simulink model "motor"  (Simulink 8.6)
settings: Solver=FixedStepDiscrete  StartTime=0.0  StopTime=inf  FixedStep=0.002  RelTol=1e-3
PostLoadFcn:
  | ,try, rti_mdl_postloadfcn(bdroot, 'UpdateModel', 160, 'rti1104'); catch, disp(lasterr); end,
undefined symbols (not defined in the file): DiscIntNeverNeededParam
(part 2 of 3)

== system motor/Chart/Open_Motor/sudu_PI ==
  In_ZV : Inport
  Discrete-Time Integrator : DiscreteIntegrator  ExternalReset=either  SampleTime=-1  SaturateOnIntegerOverflow=on  LimitOutput=on  UpperSaturationLimit=1000  LowerSaturationLimit=-1000  ICPrevOutput=DiscIntNeverNeededParam  ICPrevScaledInput=DiscIntNeverNeededParam
  Discrete-Time Integrator1 : DiscreteIntegrator  InitialConditionSetting=State (most efficient)  SampleTime=-1  ICPrevOutput=DiscIntNeverNeededParam  ICPrevScaledInput=DiscIntNeverNeededParam
  KD_KG : Gain  Gain=0
  KG_clc : DataStoreRead  DataStoreName=KG_clc
  Saturation : Saturate  UpperLimit=300  LowerLimit=-300
  Sum : Sum  Inputs=|+-
  Sum2 : Sum  Inputs=|+++
  ZV_KD : Gain  Gain=0.095
  ZV_KN : Gain  Gain=100
  ZV_Ki : Gain  Gain=0
  ZV_Kp : Gain  Gain=0.7
  ZV_Kp1 : Gain  Gain=0.001
  ZV_Kpt : Gain
  Out_ZV : Outport
  wires:
  ZV_Kpt/1 -> Sum2/2
  Discrete-Time Integrator/1 -> Sum2/1
  In_ZV/1 -> ZV_Kp/1
  ZV_Kp/1 -> ZV_Ki/1, ZV_Kp1/1, ZV_Kpt/1
  Sum2/1 -> Out_ZV/1
  ZV_Kp1/1 -> ZV_KD/1
  ZV_KD/1 -> Sum/1
  Sum/1 -> ZV_KN/1
  Discrete-Time Integrator1/1 -> Sum/2
  ZV_KN/1 -> Saturation/1, Discrete-Time Integrator1/1
  Saturation/1 -> KD_KG/1
  KD_KG/1 -> Sum2/3
  KG_clc/1 -> Discrete-Time Integrator/2
  ZV_Ki/1 -> Discrete-Time Integrator/1

== system motor/Chart/Showing/If Action Subsystem1 ==
  Action Port : ActionPort  ActionType=then
  Data Store Write : DataStoreWrite  DataStoreName=Angle_S
  Sine Wave : Sin  Frequency=pi/3
  wires:
  Sine Wave/1 -> Data Store Write/1

== system motor/Chart/Showing/If Action Subsystem2 ==
  Action Port : ActionPort  ActionType=elseif
  Data Store Write : DataStoreWrite  DataStoreName=Angle_S
  Sine Wave : Sin  Frequency=pi/4
  wires:
  Sine Wave/1 -> Data Store Write/1

== system motor/Chart/Showing/If Action Subsystem3 ==
  Action Port : ActionPort  ActionType=then
  Data Store Write : DataStoreWrite  DataStoreName=Angle_S
  Sine Wave : Sin  Frequency=pi/5
  wires:
  Sine Wave/1 -> Data Store Write/1

== system motor/Chart/Showing/If Action Subsystem4 ==
  Action Port : ActionPort  ActionType=elseif
  Data Store Write : DataStoreWrite  DataStoreName=Angle_S
  Sine Wave : Sin  Frequency=pi/6
  wires:
  Sine Wave/1 -> Data Store Write/1

== system motor/Chart/Showing/If Action Subsystem5 ==
  Action Port : ActionPort  ActionType=then
  Data Store Write : DataStoreWrite  DataStoreName=Angle_S
  Sine Wave : Sin  Frequency=pi/8
  wires:
  Sine Wave/1 -> Data Store Write/1

== system motor/Chart/Showing/If Action Subsystem6 ==
  Action Port : ActionPort  ActionType=elseif
  Data Store Write : DataStoreWrite  DataStoreName=Angle_S
  Sine Wave : Sin  Frequency=pi/10
  wires:
  Sine Wave/1 -> Data Store Write/1

== system motor/Chart/Showing/If Action Subsystem7 ==
  Action Port : ActionPort  ActionType=then
  Data Store Write : DataStoreWrite  DataStoreName=Angle_S
  Sine Wave : Sin  Frequency=pi/13
  wires:
  Sine Wave/1 -> Data Store Write/1

== system motor/Chart/Showing/If Action Subsystem8 ==
  Action Port : ActionPort  ActionType=elseif
  Data Store Write : DataStoreWrite  DataStoreName=Angle_S
  Sine Wave : Sin  Frequency=pi/15
  wires:
  Sine Wave/1 -> Data Store Write/1

== system motor/Chart/Angle_Calculation/If Action Subsystem1/ZYDX_HYDG ==
  l2 : Inport
  Cl1 : Fcn  Expr=(2*0.1*0.1+0.2655*0.2655-u*u)/(2*0.1*0.1)
  Fcn : Fcn  Expr=(2.655-sqrt(2.655*2.655-u*u+1))/(u+1)
  Fcn4 : Fcn  Expr=2*atan(u)
  Fcn7 : Fcn  Expr=u+0.2655
  x : Outport
  wires:
  Fcn4/1 -> x/1
  l2/1 -> Fcn7/1
  Fcn/1 -> Fcn4/1
  Fcn7/1 -> Cl1/1
  Cl1/1 -> Fcn/1

== system motor/Chart/Angle_Calculation/If Action Subsystem2/ZYDX_XHZY ==
  Zl : Inport
  Fcn1 : Fcn  Expr=u+265.5
  Fcn2 : Fcn  Expr=(90490.25-u*u)/(20000)
  Fcn3 : Fcn  Expr=(2.655-sqrt(2.655*2.655-u*u+1))/(u+1)
  Fcn6 : Fcn  Expr=2*atan(u)
  Zq : Outport
  wires:
  Fcn3/1 -> Fcn6/1
  Zl/1 -> Fcn1/1
  Fcn6/1 -> Zq/1
  Fcn1/1 -> Fcn2/1
  Fcn2/1 -> Fcn3/1

== system motor/Chart/Angle_Calculation/If Action Subsystem3/ZYDX_XHHY ==
  Hl : Inport  OutDataTypeStr=double
  Zl : Inport  Port=2  OutDataTypeStr=double
  Fcn1 : Fcn  Expr=u+265.5
  Fcn10 : Fcn  Expr=u*u+1
  Fcn11 : Fcn  Expr=sqrt(u)
  Fcn12 : Fcn  Expr=2*atan(u)
  Fcn2 : Fcn  Expr=(90490.25-u*u)/(20000)
  Fcn3 : Fcn  Expr=(2.655-sqrt(2.655*2.655-u*u+1))/(u+1)
  Fcn4 : Fcn  Expr=2.655*cos(u)
  Fcn5 : Fcn  Expr=u+265.5
  Fcn6 : Fcn  Expr=2*atan(u)
  Fcn7 : Fcn  Expr=(90490.25-u*u)/(20000)
  Fcn8 : Fcn  Expr=u*u
  Fcn9 : Fcn  Expr=1/(u+1)
  Product : Product  RndMeth=Zero
  Sum2 : Sum  Inputs=|+-
  Sum3 : Sum  Inputs=|+-
  Hq : Outport
  wires:
  Fcn11/1 -> Sum2/2
  Fcn4/1 -> Fcn10/1, Sum2/1
  Fcn3/1 -> Fcn6/1
  Hl/1 -> Fcn5/1
  Fcn1/1 -> Fcn2/1
  Product/1 -> Fcn12/1
  Fcn12/1 -> Hq/1
  Fcn2/1 -> Fcn3/1
  Fcn7/1 -> Fcn9/1, Fcn8/1
  Fcn6/1 -> Fcn4/1
  Zl/1 -> Fcn1/1
  Sum2/1 -> Product/1
  Fcn10/1 -> Sum3/1
  Fcn5/1 -> Fcn7/1
  Sum3/1 -> Fcn11/1
  Fcn9/1 -> Product/2
  Fcn8/1 -> Sum3/2

== system motor/Chart/Angle_Calculation_HY/fs_plat/ZYDX_HYDG ==
  l2 : Inport
  Cl1 : Fcn  Expr=(2*0.1*0.1+0.2655*0.2655-u*u)/(2*0.1*0.1)
  Fcn : Fcn  Expr=(2.655-sqrt(2.655*2.655-u*u+1))/(u+1)
  Fcn4 : Fcn  Expr=2*atan(u)
  Fcn7 : Fcn  Expr=u+0.2655
  x : Outport
  wires:
  Fcn4/1 -> x/1
  l2/1 -> Fcn7/1
  Fcn/1 -> Fcn4/1
  Fcn7/1 -> Cl1/1
  Cl1/1 -> Fcn/1

== system motor/Chart/BJ/If Action Subsystem/If Action Subsystem ==
  Action Port : ActionPort  ActionType=then
  Data Store Write : DataStoreWrite  DataStoreName=PC1
  Data Store Write1 : DataStoreWrite  DataStoreName=PC2
  Data Type Conversion : DataTypeConversion  OutDataTypeStr=boolean
  Pulse Generator : DiscretePulseGenerator  Period=500  PulseWidth=250  SampleTime=-1
  wires:
  Pulse Generator/1 -> Data Type Conversion/1
  Data Type Conversion/1 -> Data Store Write1/1, Data Store Write/1

== system motor/Chart/BJ/If Action Subsystem/If Action Subsystem1 ==
  Action Port : ActionPort  ActionType=elseif
  Constant : Constant  OutDataTypeStr=boolean
  Data Store Write : DataStoreWrite  DataStoreName=PC1
  Data Store Write1 : DataStoreWrite  DataStoreName=PC2
  Data Type Conversion : DataTypeConversion  OutDataTypeStr=boolean
  Pulse Generator : DiscretePulseGenerator  Period=500  PulseWidth=250  SampleTime=-1
  wires:
  Pulse Generator/1 -> Data Type Conversion/1
  Data Type Conversion/1 -> Data Store Write/1
  Constant/1 -> Data Store Write1/1

== system motor/Chart/BJ/If Action Subsystem/If Action Subsystem2 ==
  Action Port : ActionPort  ActionType=else
  Constant : Constant  OutDataTypeStr=boolean
  Constant1 : Constant  Value=0  OutDataTypeStr=boolean
  Data Store Write : DataStoreWrite  DataStoreName=PC1
  Data Store Write1 : DataStoreWrite  DataStoreName=PC2
  wires:
  Constant/1 -> Data Store Write/1
  Constant1/1 -> Data Store Write1/1

== system motor/Chart/BJ/If Action Subsystem1/If Action Subsystem ==
  Action Port : ActionPort  ActionType=then
  Data Store Write : DataStoreWrite  DataStoreName=PC1
  Data Store Write1 : DataStoreWrite  DataStoreName=PC2
  Data Type Conversion : DataTypeConversion  OutDataTypeStr=boolean
  Pulse Generator : DiscretePulseGenerator  Period=500  PulseWidth=250  SampleTime=-1
  wires:
  Pulse Generator/1 -> Data Type Conversion/1
  Data Type Conversion/1 -> Data Store Write1/1, Data Store Write/1

== system motor/Chart/BJ/If Action Subsystem1/If Action Subsystem1 ==
  Action Port : ActionPort  ActionType=elseif
  Constant : Constant  OutDataTypeStr=boolean
  Data Store Write : DataStoreWrite  DataStoreName=PC1
  Data Store Write1 : DataStoreWrite  DataStoreName=PC2
  Data Type Conversion : DataTypeConversion  OutDataTypeStr=boolean
  Pulse Generator : DiscretePulseGenerator  Period=500  PulseWidth=250  SampleTime=-1
  wires:
  Pulse Generator/1 -> Data Type Conversion/1
  Data Type Conversion/1 -> Data Store Write/1
  Constant/1 -> Data Store Write1/1

== system motor/Chart/BJ/If Action Subsystem1/If Action Subsystem2 ==
  Action Port : ActionPort  ActionType=else
  Constant : Constant  OutDataTypeStr=boolean
  Data Store Write : DataStoreWrite  DataStoreName=PC2
  Data Store Write1 : DataStoreWrite  DataStoreName=PC1
  Data Type Conversion : DataTypeConversion  OutDataTypeStr=boolean
  Pulse Generator : DiscretePulseGenerator  Period=500  PulseWidth=250  SampleTime=-1
  wires:
  Pulse Generator/1 -> Data Type Conversion/1
  Data Type Conversion/1 -> Data Store Write/1
  Constant/1 -> Data Store Write1/1

== system motor/Chart/BJ/If Action Subsystem2/If Action Subsystem ==
  Action Port : ActionPort  ActionType=then
  Data Store Write : DataStoreWrite  DataStoreName=PC1
  Data Store Write1 : DataStoreWrite  DataStoreName=PC2
  Data Type Conversion : DataTypeConversion  OutDataTypeStr=boolean
  Pulse Generator : DiscretePulseGenerator  Period=500  PulseWidth=250  SampleTime=-1
  wires:
  Pulse Generator/1 -> Data Type Conversion/1
  Data Type Conversion/1 -> Data Store Write1/1, Data Store Write/1

== system motor/Chart/BJ/If Action Subsystem2/If Action Subsystem1 ==
  Action Port : ActionPort  ActionType=elseif
  Constant : Constant  OutDataTypeStr=boolean
  Data Store Write : DataStoreWrite  DataStoreName=PC1
  Data Store Write1 : DataStoreWrite  DataStoreName=PC2
  Data Type Conversion : DataTypeConversion  OutDataTypeStr=boolean
  Pulse Generator : DiscretePulseGenerator  Period=500  PulseWidth=250  SampleTime=-1
  wires:
  Pulse Generator/1 -> Data Type Conversion/1
  Data Type Conversion/1 -> Data Store Write/1
  Constant/1 -> Data Store Write1/1

== system motor/Chart/BJ/If Action Subsystem2/If Action Subsystem2 ==
  Action Port : ActionPort  ActionType=else
  Constant : Constant  OutDataTypeStr=boolean
  Constant1 : Constant  Value=0  OutDataTypeStr=boolean
  Data Store Write : DataStoreWrite  DataStoreName=PC1
  Data Store Write1 : DataStoreWrite  DataStoreName=PC2
  wires:
  Constant/1 -> Data Store Write/1
  Constant1/1 -> Data Store Write1/1

== system motor/Chart/Motor_HYDG/fs_plat/ZYDX_HYDG ==
  l2 : Inport
  Cl1 : Fcn  Expr=(2*0.1*0.1+0.2655*0.2655-u*u)/(2*0.1*0.1)
  Fcn : Fcn  Expr=(2.655-sqrt(2.655*2.655-u*u+1))/(u+1)
  Fcn4 : Fcn  Expr=2*atan(u)
  Fcn7 : Fcn  Expr=u+0.2655
  x : Outport
  wires:
  Fcn4/1 -> x/1
  l2/1 -> Fcn7/1
  Fcn/1 -> Fcn4/1
  Fcn7/1 -> Cl1/1
  Cl1/1 -> Fcn/1
